simulink model "bit32mul"  (R2020a)
settings: Solver=VariableStepAuto  StartTime=0.0  StopTime=10.0  RelTol=1e-3
(part 37 of 50)

== system bit32mul/Subsystem1/Subsystem/Subsystem6/Subsystem/Subsystem5 ==
  In1 : Inport
  In2 : Inport  Port=2
  In3 : Inport  Port=3
  Logical Operator2 : Logic  Operator=XOR  AllPortsSameDT=off  OutDataTypeStr=boolean
  Logical Operator3 : Logic  Operator=XOR  AllPortsSameDT=off  OutDataTypeStr=boolean
  Out1 : Outport
  wires:
  In3/1 -> Logical Operator3/2
  In2/1 -> Logical Operator2/2
  In1/1 -> Logical Operator2/1
  Logical Operator2/1 -> Logical Operator3/1
  Logical Operator3/1 -> Out1/1

== system bit32mul/Subsystem1/Subsystem/Subsystem6/Subsystem/Subsystem6 ==
  In1 : Inport
  In2 : Inport  Port=2
  Logical Operator : Logic  Operator=XOR  AllPortsSameDT=off  OutDataTypeStr=boolean
  Logical Operator1 : Logic  AllPortsSameDT=off  OutDataTypeStr=boolean
  Out1 : Outport
  Out2 : Outport  Port=2
  wires:
  In1/1 -> Logical Operator1/1, Logical Operator/1
  Logical Operator1/1 -> Out2/1
  In2/1 -> Logical Operator1/2, Logical Operator/2
  Logical Operator/1 -> Out1/1

== system bit32mul/Subsystem1/Subsystem/Subsystem6/Subsystem/Subsystem7 ==
  In1 : Inport
  In2 : Inport  Port=2
  In3 : Inport  Port=3
  Logical Operator2 : Logic  Operator=XOR  AllPortsSameDT=off  OutDataTypeStr=boolean
  Logical Operator3 : Logic  Operator=XOR  AllPortsSameDT=off  OutDataTypeStr=boolean
  Out1 : Outport
  wires:
  In3/1 -> Logical Operator3/2
  In2/1 -> Logical Operator2/2
  In1/1 -> Logical Operator2/1
  Logical Operator2/1 -> Logical Operator3/1
  Logical Operator3/1 -> Out1/1

== system bit32mul/Subsystem1/Subsystem/Subsystem6/Subsystem/Subsystem8 ==
  In1 : Inport
  In2 : Inport  Port=2
  Logical Operator : Logic  Operator=XOR  AllPortsSameDT=off  OutDataTypeStr=boolean
  Logical Operator1 : Logic  AllPortsSameDT=off  OutDataTypeStr=boolean
  Out1 : Outport
  Out2 : Outport  Port=2
  wires:
  In1/1 -> Logical Operator1/1, Logical Operator/1
  Logical Operator1/1 -> Out2/1
  In2/1 -> Logical Operator1/2, Logical Operator/2
  Logical Operator/1 -> Out1/1

== system bit32mul/Subsystem1/Subsystem/Subsystem6/Subsystem4/Subsystem1 ==
  In1 : Inport
  In2 : Inport  Port=2
  Logical Operator : Logic  Operator=XOR  AllPortsSameDT=off  OutDataTypeStr=boolean
  Logical Operator1 : Logic  AllPortsSameDT=off  OutDataTypeStr=boolean
  Out1 : Outport
  Out2 : Outport  Port=2
  wires:
  In1/1 -> Logical Operator1/1, Logical Operator/1
  Logical Operator1/1 -> Out2/1
  In2/1 -> Logical Operator1/2, Logical Operator/2
  Logical Operator/1 -> Out1/1

== system bit32mul/Subsystem1/Subsystem/Subsystem6/Subsystem4/Subsystem2 ==
  In1 : Inport
  In2 : Inport  Port=2
  In3 : Inport  Port=3
  Logical Operator2 : Logic  Operator=XOR  AllPortsSameDT=off  OutDataTypeStr=boolean
  Logical Operator3 : Logic  Operator=XOR  AllPortsSameDT=off  OutDataTypeStr=boolean
  Out1 : Outport
  wires:
  In3/1 -> Logical Operator3/2
  In2/1 -> Logical Operator2/2
  In1/1 -> Logical Operator2/1
  Logical Operator2/1 -> Logical Operator3/1
  Logical Operator3/1 -> Out1/1

== system bit32mul/Subsystem1/Subsystem/Subsystem6/Subsystem4/Subsystem3 ==
  In1 : Inport
  In2 : Inport  Port=2
  In3 : Inport  Port=3
  Logical Operator2 : Logic  Operator=XOR  AllPortsSameDT=off  OutDataTypeStr=boolean
  Logical Operator3 : Logic  Operator=XOR  AllPortsSameDT=off  OutDataTypeStr=boolean
  Out1 : Outport
  wires:
  In3/1 -> Logical Operator3/2
  In2/1 -> Logical Operator2/2
  In1/1 -> Logical Operator2/1
  Logical Operator2/1 -> Logical Operator3/1
  Logical Operator3/1 -> Out1/1

== system bit32mul/Subsystem1/Subsystem/Subsystem6/Subsystem4/Subsystem4 ==
  In1 : Inport
  In2 : Inport  Port=2
  Logical Operator : Logic  Operator=XOR  AllPortsSameDT=off  OutDataTypeStr=boolean
  Logical Operator1 : Logic  AllPortsSameDT=off  OutDataTypeStr=boolean
  Out1 : Outport
  Out2 : Outport  Port=2
  wires:
  In1/1 -> Logical Operator1/1, Logical Operator/1
  Logical Operator1/1 -> Out2/1
  In2/1 -> Logical Operator1/2, Logical Operator/2
  Logical Operator/1 -> Out1/1

== system bit32mul/Subsystem1/Subsystem/Subsystem6/Subsystem4/Subsystem5 ==
  In1 : Inport
  In2 : Inport  Port=2
  In3 : Inport  Port=3
  Logical Operator2 : Logic  Operator=XOR  AllPortsSameDT=off  OutDataTypeStr=boolean
  Logical Operator3 : Logic  Operator=XOR  AllPortsSameDT=off  OutDataTypeStr=boolean
  Out1 : Outport
  wires:
  In3/1 -> Logical Operator3/2
  In2/1 -> Logical Operator2/2
  In1/1 -> Logical Operator2/1
  Logical Operator2/1 -> Logical Operator3/1
  Logical Operator3/1 -> Out1/1

== system bit32mul/Subsystem1/Subsystem/Subsystem6/Subsystem4/Subsystem6 ==
  In1 : Inport
  In2 : Inport  Port=2
  Logical Operator : Logic  Operator=XOR  AllPortsSameDT=off  OutDataTypeStr=boolean
  Logical Operator1 : Logic  AllPortsSameDT=off  OutDataTypeStr=boolean
  Out1 : Outport
  Out2 : Outport  Port=2
  wires:
  In1/1 -> Logical Operator1/1, Logical Operator/1
  Logical Operator1/1 -> Out2/1
  In2/1 -> Logical Operator1/2, Logical Operator/2
  Logical Operator/1 -> Out1/1

== system bit32mul/Subsystem1/Subsystem/Subsystem6/Subsystem4/Subsystem7 ==
  In1 : Inport
  In2 : Inport  Port=2
  In3 : Inport  Port=3
  Logical Operator2 : Logic  Operator=XOR  AllPortsSameDT=off  OutDataTypeStr=boolean
  Logical Operator3 : Logic  Operator=XOR  AllPortsSameDT=off  OutDataTypeStr=boolean
  Out1 : Outport
  wires:
  In3/1 -> Logical Operator3/2
  In2/1 -> Logical Operator2/2
  In1/1 -> Logical Operator2/1
  Logical Operator2/1 -> Logical Operator3/1
  Logical Operator3/1 -> Out1/1

== system bit32mul/Subsystem1/Subsystem/Subsystem6/Subsystem4/Subsystem8 ==
  In1 : Inport
  In2 : Inport  Port=2
  Logical Operator : Logic  Operator=XOR  AllPortsSameDT=off  OutDataTypeStr=boolean
  Logical Operator1 : Logic  AllPortsSameDT=off  OutDataTypeStr=boolean
  Out1 : Outport
  Out2 : Outport  Port=2
  wires:
  In1/1 -> Logical Operator1/1, Logical Operator/1
  Logical Operator1/1 -> Out2/1
  In2/1 -> Logical Operator1/2, Logical Operator/2
  Logical Operator/1 -> Out1/1

== system bit32mul/Subsystem1/Subsystem1/Subsystem4/Subsystem/Subsystem1 ==
  In1 : Inport
  In2 : Inport  Port=2
  Logical Operator : Logic  Operator=XOR  AllPortsSameDT=off  OutDataTypeStr=boolean
  Logical Operator1 : Logic  AllPortsSameDT=off  OutDataTypeStr=boolean
  Out1 : Outport
  Out2 : Outport  Port=2
  wires:
  In1/1 -> Logical Operator1/1, Logical Operator/1
  Logical Operator1/1 -> Out2/1
  In2/1 -> Logical Operator1/2, Logical Operator/2
  Logical Operator/1 -> Out1/1

== system bit32mul/Subsystem1/Subsystem1/Subsystem4/Subsystem/Subsystem2 ==
  In1 : Inport
  In2 : Inport  Port=2
  In3 : Inport  Port=3
  Logical Operator2 : Logic  Operator=XOR  AllPortsSameDT=off  OutDataTypeStr=boolean
  Logical Operator3 : Logic  Operator=XOR  AllPortsSameDT=off  OutDataTypeStr=boolean
  Out1 : Outport
  wires:
  In3/1 -> Logical Operator3/2
  In2/1 -> Logical Operator2/2
  In1/1 -> Logical Operator2/1
  Logical Operator2/1 -> Logical Operator3/1
  Logical Operator3/1 -> Out1/1

== system bit32mul/Subsystem1/Subsystem1/Subsystem4/Subsystem/Subsystem3 ==
  In1 : Inport
  In2 : Inport  Port=2
  In3 : Inport  Port=3
  Logical Operator2 : Logic  Operator=XOR  AllPortsSameDT=off  OutDataTypeStr=boolean
  Logical Operator3 : Logic  Operator=XOR  AllPortsSameDT=off  OutDataTypeStr=boolean
  Out1 : Outport
  wires:
  In3/1 -> Logical Operator3/2
  In2/1 -> Logical Operator2/2
  In1/1 -> Logical Operator2/1
  Logical Operator2/1 -> Logical Operator3/1
  Logical Operator3/1 -> Out1/1

== system bit32mul/Subsystem1/Subsystem1/Subsystem4/Subsystem/Subsystem4 ==
  In1 : Inport
  In2 : Inport  Port=2
  Logical Operator : Logic  Operator=XOR  AllPortsSameDT=off  OutDataTypeStr=boolean
  Logical Operator1 : Logic  AllPortsSameDT=off  OutDataTypeStr=boolean
  Out1 : Outport
  Out2 : Outport  Port=2
  wires:
  In1/1 -> Logical Operator1/1, Logical Operator/1
  Logical Operator1/1 -> Out2/1
  In2/1 -> Logical Operator1/2, Logical Operator/2
  Logical Operator/1 -> Out1/1

== system bit32mul/Subsystem1/Subsystem1/Subsystem4/Subsystem/Subsystem5 ==
  In1 : Inport
  In2 : Inport  Port=2
  In3 : Inport  Port=3
  Logical Operator2 : Logic  Operator=XOR  AllPortsSameDT=off  OutDataTypeStr=boolean
  Logical Operator3 : Logic  Operator=XOR  AllPortsSameDT=off  OutDataTypeStr=boolean
  Out1 : Outport
  wires:
  In3/1 -> Logical Operator3/2
  In2/1 -> Logical Operator2/2
  In1/1 -> Logical Operator2/1
  Logical Operator2/1 -> Logical Operator3/1
  Logical Operator3/1 -> Out1/1

== system bit32mul/Subsystem1/Subsystem1/Subsystem4/Subsystem/Subsystem6 ==
  In1 : Inport
  In2 : Inport  Port=2
  Logical Operator : Logic  Operator=XOR  AllPortsSameDT=off  OutDataTypeStr=boolean
  Logical Operator1 : Logic  AllPortsSameDT=off  OutDataTypeStr=boolean
  Out1 : Outport
  Out2 : Outport  Port=2
  wires:
  In1/1 -> Logical Operator1/1, Logical Operator/1
  Logical Operator1/1 -> Out2/1
  In2/1 -> Logical Operator1/2, Logical Operator/2
  Logical Operator/1 -> Out1/1

== system bit32mul/Subsystem1/Subsystem1/Subsystem4/Subsystem/Subsystem7 ==
  In1 : Inport
  In2 : Inport  Port=2
  In3 : Inport  Port=3
  Logical Operator2 : Logic  Operator=XOR  AllPortsSameDT=off  OutDataTypeStr=boolean
  Logical Operator3 : Logic  Operator=XOR  AllPortsSameDT=off  OutDataTypeStr=boolean
  Out1 : Outport
  wires:
  In3/1 -> Logical Operator3/2
  In2/1 -> Logical Operator2/2
  In1/1 -> Logical Operator2/1
  Logical Operator2/1 -> Logical Operator3/1
  Logical Operator3/1 -> Out1/1

== system bit32mul/Subsystem1/Subsystem1/Subsystem4/Subsystem/Subsystem8 ==
  In1 : Inport
  In2 : Inport  Port=2
  Logical Operator : Logic  Operator=XOR  AllPortsSameDT=off  OutDataTypeStr=boolean
  Logical Operator1 : Logic  AllPortsSameDT=off  OutDataTypeStr=boolean
  Out1 : Outport
  Out2 : Outport  Port=2
  wires:
  In1/1 -> Logical Operator1/1, Logical Operator/1
  Logical Operator1/1 -> Out2/1
  In2/1 -> Logical Operator1/2, Logical Operator/2
  Logical Operator/1 -> Out1/1

== system bit32mul/Subsystem1/Subsystem1/Subsystem4/Subsystem4/Subsystem1 ==
  In1 : Inport
  In2 : Inport  Port=2
  Logical Operator : Logic  Operator=XOR  AllPortsSameDT=off  OutDataTypeStr=boolean
  Logical Operator1 : Logic  AllPortsSameDT=off  OutDataTypeStr=boolean
  Out1 : Outport
  Out2 : Outport  Port=2
  wires:
  In1/1 -> Logical Operator1/1, Logical Operator/1
  Logical Operator1/1 -> Out2/1
  In2/1 -> Logical Operator1/2, Logical Operator/2
  Logical Operator/1 -> Out1/1

== system bit32mul/Subsystem1/Subsystem1/Subsystem4/Subsystem4/Subsystem2 ==
  In1 : Inport
  In2 : Inport  Port=2
  In3 : Inport  Port=3
  Logical Operator2 : Logic  Operator=XOR  AllPortsSameDT=off  OutDataTypeStr=boolean
  Logical Operator3 : Logic  Operator=XOR  AllPortsSameDT=off  OutDataTypeStr=boolean
  Out1 : Outport
  wires:
  In3/1 -> Logical Operator3/2
  In2/1 -> Logical Operator2/2
  In1/1 -> Logical Operator2/1
  Logical Operator2/1 -> Logical Operator3/1
  Logical Operator3/1 -> Out1/1

== system bit32mul/Subsystem1/Subsystem1/Subsystem4/Subsystem4/Subsystem3 ==
  In1 : Inport
  In2 : Inport  Port=2
  In3 : Inport  Port=3
  Logical Operator2 : Logic  Operator=XOR  AllPortsSameDT=off  OutDataTypeStr=boolean
  Logical Operator3 : Logic  Operator=XOR  AllPortsSameDT=off  OutDataTypeStr=boolean
  Out1 : Outport
  wires:
  In3/1 -> Logical Operator3/2
  In2/1 -> Logical Operator2/2
  In1/1 -> Logical Operator2/1
  Logical Operator2/1 -> Logical Operator3/1
  Logical Operator3/1 -> Out1/1

== system bit32mul/Subsystem1/Subsystem1/Subsystem4/Subsystem4/Subsystem4 ==
  In1 : Inport
  In2 : Inport  Port=2
  Logical Operator : Logic  Operator=XOR  AllPortsSameDT=off  OutDataTypeStr=boolean
  Logical Operator1 : Logic  AllPortsSameDT=off  OutDataTypeStr=boolean
  Out1 : Outport
  Out2 : Outport  Port=2
  wires:
  In1/1 -> Logical Operator1/1, Logical Operator/1
  Logical Operator1/1 -> Out2/1
  In2/1 -> Logical Operator1/2, Logical Operator/2
  Logical Operator/1 -> Out1/1

== system bit32mul/Subsystem1/Subsystem1/Subsystem4/Subsystem4/Subsystem5 ==
  In1 : Inport
  In2 : Inport  Port=2
  In3 : Inport  Port=3
  Logical Operator2 : Logic  Operator=XOR  AllPortsSameDT=off  OutDataTypeStr=boolean
  Logical Operator3 : Logic  Operator=XOR  AllPortsSameDT=off  OutDataTypeStr=boolean
  Out1 : Outport
  wires:
  In3/1 -> Logical Operator3/2
  In2/1 -> Logical Operator2/2
  In1/1 -> Logical Operator2/1
  Logical Operator2/1 -> Logical Operator3/1
  Logical Operator3/1 -> Out1/1

== system bit32mul/Subsystem1/Subsystem1/Subsystem4/Subsystem4/Subsystem6 ==
  In1 : Inport
  In2 : Inport  Port=2
  Logical Operator : Logic  Operator=XOR  AllPortsSameDT=off  OutDataTypeStr=boolean
  Logical Operator1 : Logic  AllPortsSameDT=off  OutDataTypeStr=boolean
  Out1 : Outport
  Out2 : Outport  Port=2
  wires:
  In1/1 -> Logical Operator1/1, Logical Operator/1
  Logical Operator1/1 -> Out2/1
  In2/1 -> Logical Operator1/2, Logical Operator/2
  Logical Operator/1 -> Out1/1

== system bit32mul/Subsystem1/Subsystem1/Subsystem4/Subsystem4/Subsystem7 ==
  In1 : Inport
  In2 : Inport  Port=2
  In3 : Inport  Port=3
  Logical Operator2 : Logic  Operator=XOR  AllPortsSameDT=off  OutDataTypeStr=boolean
  Logical Operator3 : Logic  Operator=XOR  AllPortsSameDT=off  OutDataTypeStr=boolean
  Out1 : Outport
  wires:
  In3/1 -> Logical Operator3/2
  In2/1 -> Logical Operator2/2
  In1/1 -> Logical Operator2/1
  Logical Operator2/1 -> Logical Operator3/1
  Logical Operator3/1 -> Out1/1

== system bit32mul/Subsystem1/Subsystem1/Subsystem4/Subsystem4/Subsystem8 ==
  In1 : Inport
  In2 : Inport  Port=2
  Logical Operator : Logic  Operator=XOR  AllPortsSameDT=off  OutDataTypeStr=boolean
  Logical Operator1 : Logic  AllPortsSameDT=off  OutDataTypeStr=boolean
  Out1 : Outport
  Out2 : Outport  Port=2
  wires:
  In1/1 -> Logical Operator1/1, Logical Operator/1
  Logical Operator1/1 -> Out2/1
  In2/1 -> Logical Operator1/2, Logical Operator/2
  Logical Operator/1 -> Out1/1

== system bit32mul/Subsystem1/Subsystem1/Subsystem5/Subsystem/Subsystem1 ==
  In1 : Inport
  In2 : Inport  Port=2
  Logical Operator : Logic  Operator=XOR  AllPortsSameDT=off  OutDataTypeStr=boolean
  Logical Operator1 : Logic  AllPortsSameDT=off  OutDataTypeStr=boolean
  Out1 : Outport
  Out2 : Outport  Port=2
  wires:
  In1/1 -> Logical Operator1/1, Logical Operator/1
  Logical Operator1/1 -> Out2/1
  In2/1 -> Logical Operator1/2, Logical Operator/2
  Logical Operator/1 -> Out1/1

== system bit32mul/Subsystem1/Subsystem1/Subsystem5/Subsystem/Subsystem2 ==
  In1 : Inport
  In2 : Inport  Port=2
  In3 : Inport  Port=3
  Logical Operator2 : Logic  Operator=XOR  AllPortsSameDT=off  OutDataTypeStr=boolean
  Logical Operator3 : Logic  Operator=XOR  AllPortsSameDT=off  OutDataTypeStr=boolean
  Out1 : Outport
  wires:
  In3/1 -> Logical Operator3/2
  In2/1 -> Logical Operator2/2
  In1/1 -> Logical Operator2/1
  Logical Operator2/1 -> Logical Operator3/1
  Logical Operator3/1 -> Out1/1

== system bit32mul/Subsystem1/Subsystem1/Subsystem5/Subsystem/Subsystem3 ==
  In1 : Inport
  In2 : Inport  Port=2
  In3 : Inport  Port=3
  Logical Operator2 : Logic  Operator=XOR  AllPortsSameDT=off  OutDataTypeStr=boolean
  Logical Operator3 : Logic  Operator=XOR  AllPortsSameDT=off  OutDataTypeStr=boolean
  Out1 : Outport
  wires:
  In3/1 -> Logical Operator3/2
  In2/1 -> Logical Operator2/2
  In1/1 -> Logical Operator2/1
  Logical Operator2/1 -> Logical Operator3/1
  Logical Operator3/1 -> Out1/1

== system bit32mul/Subsystem1/Subsystem1/Subsystem5/Subsystem/Subsystem4 ==
  In1 : Inport
  In2 : Inport  Port=2
  Logical Operator : Logic  Operator=XOR  AllPortsSameDT=off  OutDataTypeStr=boolean
  Logical Operator1 : Logic  AllPortsSameDT=off  OutDataTypeStr=boolean
  Out1 : Outport
  Out2 : Outport  Port=2
  wires:
  In1/1 -> Logical Operator1/1, Logical Operator/1
  Logical Operator1/1 -> Out2/1
  In2/1 -> Logical Operator1/2, Logical Operator/2
  Logical Operator/1 -> Out1/1

== system bit32mul/Subsystem1/Subsystem1/Subsystem5/Subsystem/Subsystem5 ==
  In1 : Inport
  In2 : Inport  Port=2
  In3 : Inport  Port=3
  Logical Operator2 : Logic  Operator=XOR  AllPortsSameDT=off  OutDataTypeStr=boolean
  Logical Operator3 : Logic  Operator=XOR  AllPortsSameDT=off  OutDataTypeStr=boolean
  Out1 : Outport
  wires:
  In3/1 -> Logical Operator3/2
  In2/1 -> Logical Operator2/2
  In1/1 -> Logical Operator2/1
  Logical Operator2/1 -> Logical Operator3/1
  Logical Operator3/1 -> Out1/1

== system bit32mul/Subsystem1/Subsystem1/Subsystem5/Subsystem/Subsystem6 ==
  In1 : Inport
  In2 : Inport  Port=2
  Logical Operator : Logic  Operator=XOR  AllPortsSameDT=off  OutDataTypeStr=boolean
  Logical Operator1 : Logic  AllPortsSameDT=off  OutDataTypeStr=boolean
  Out1 : Outport
  Out2 : Outport  Port=2
  wires:
  In1/1 -> Logical Operator1/1, Logical Operator/1
  Logical Operator1/1 -> Out2/1
  In2/1 -> Logical Operator1/2, Logical Operator/2
  Logical Operator/1 -> Out1/1

== system bit32mul/Subsystem1/Subsystem1/Subsystem5/Subsystem/Subsystem7 ==
  In1 : Inport
  In2 : Inport  Port=2
  In3 : Inport  Port=3
  Logical Operator2 : Logic  Operator=XOR  AllPortsSameDT=off  OutDataTypeStr=boolean
  Logical Operator3 : Logic  Operator=XOR  AllPortsSameDT=off  OutDataTypeStr=boolean
  Out1 : Outport
  wires:
  In3/1 -> Logical Operator3/2
  In2/1 -> Logical Operator2/2
  In1/1 -> Logical Operator2/1
  Logical Operator2/1 -> Logical Operator3/1
  Logical Operator3/1 -> Out1/1

== system bit32mul/Subsystem1/Subsystem1/Subsystem5/Subsystem/Subsystem8 ==
  In1 : Inport
  In2 : Inport  Port=2
  Logical Operator : Logic  Operator=XOR  AllPortsSameDT=off  OutDataTypeStr=boolean
  Logical Operator1 : Logic  AllPortsSameDT=off  OutDataTypeStr=boolean
  Out1 : Outport
  Out2 : Outport  Port=2
  wires:
  In1/1 -> Logical Operator1/1, Logical Operator/1
  Logical Operator1/1 -> Out2/1
  In2/1 -> Logical Operator1/2, Logical Operator/2
  Logical Operator/1 -> Out1/1

== system bit32mul/Subsystem1/Subsystem1/Subsystem5/Subsystem4/Subsystem1 ==
  In1 : Inport
  In2 : Inport  Port=2
  Logical Operator : Logic  Operator=XOR  AllPortsSameDT=off  OutDataTypeStr=boolean
  Logical Operator1 : Logic  AllPortsSameDT=off  OutDataTypeStr=boolean
  Out1 : Outport
  Out2 : Outport  Port=2
  wires:
  In1/1 -> Logical Operator1/1, Logical Operator/1
  Logical Operator1/1 -> Out2/1
  In2/1 -> Logical Operator1/2, Logical Operator/2
  Logical Operator/1 -> Out1/1

== system bit32mul/Subsystem1/Subsystem1/Subsystem5/Subsystem4/Subsystem2 ==
  In1 : Inport
  In2 : Inport  Port=2
  In3 : Inport  Port=3
  Logical Operator2 : Logic  Operator=XOR  AllPortsSameDT=off  OutDataTypeStr=boolean
  Logical Operator3 : Logic  Operator=XOR  AllPortsSameDT=off  OutDataTypeStr=boolean
  Out1 : Outport
  wires:
  In3/1 -> Logical Operator3/2
  In2/1 -> Logical Operator2/2
  In1/1 -> Logical Operator2/1
  Logical Operator2/1 -> Logical Operator3/1
  Logical Operator3/1 -> Out1/1

== system bit32mul/Subsystem1/Subsystem1/Subsystem5/Subsystem4/Subsystem3 ==
  In1 : Inport
  In2 : Inport  Port=2
  In3 : Inport  Port=3
  Logical Operator2 : Logic  Operator=XOR  AllPortsSameDT=off  OutDataTypeStr=boolean
  Logical Operator3 : Logic  Operator=XOR  AllPortsSameDT=off  OutDataTypeStr=boolean
  Out1 : Outport
  wires:
  In3/1 -> Logical Operator3/2
  In2/1 -> Logical Operator2/2
  In1/1 -> Logical Operator2/1
  Logical Operator2/1 -> Logical Operator3/1
  Logical Operator3/1 -> Out1/1

== system bit32mul/Subsystem1/Subsystem1/Subsystem5/Subsystem4/Subsystem4 ==
  In1 : Inport
  In2 : Inport  Port=2
  Logical Operator : Logic  Operator=XOR  AllPortsSameDT=off  OutDataTypeStr=boolean
  Logical Operator1 : Logic  AllPortsSameDT=off  OutDataTypeStr=boolean
  Out1 : Outport
  Out2 : Outport  Port=2
  wires:
  In1/1 -> Logical Operator1/1, Logical Operator/1
  Logical Operator1/1 -> Out2/1
  In2/1 -> Logical Operator1/2, Logical Operator/2
  Logical Operator/1 -> Out1/1

== system bit32mul/Subsystem1/Subsystem1/Subsystem5/Subsystem4/Subsystem5 ==
  In1 : Inport
  In2 : Inport  Port=2
  In3 : Inport  Port=3
  Logical Operator2 : Logic  Operator=XOR  AllPortsSameDT=off  OutDataTypeStr=boolean
  Logical Operator3 : Logic  Operator=XOR  AllPortsSameDT=off  OutDataTypeStr=boolean
  Out1 : Outport
  wires:
  In3/1 -> Logical Operator3/2
  In2/1 -> Logical Operator2/2
  In1/1 -> Logical Operator2/1
  Logical Operator2/1 -> Logical Operator3/1
  Logical Operator3/1 -> Out1/1

== system bit32mul/Subsystem1/Subsystem1/Subsystem5/Subsystem4/Subsystem6 ==
  In1 : Inport
  In2 : Inport  Port=2
  Logical Operator : Logic  Operator=XOR  AllPortsSameDT=off  OutDataTypeStr=boolean
  Logical Operator1 : Logic  AllPortsSameDT=off  OutDataTypeStr=boolean
  Out1 : Outport
  Out2 : Outport  Port=2
  wires:
  In1/1 -> Logical Operator1/1, Logical Operator/1
  Logical Operator1/1 -> Out2/1
  In2/1 -> Logical Operator1/2, Logical Operator/2
  Logical Operator/1 -> Out1/1

== system bit32mul/Subsystem1/Subsystem1/Subsystem5/Subsystem4/Subsystem7 ==
  In1 : Inport
  In2 : Inport  Port=2
  In3 : Inport  Port=3
  Logical Operator2 : Logic  Operator=XOR  AllPortsSameDT=off  OutDataTypeStr=boolean
  Logical Operator3 : Logic  Operator=XOR  AllPortsSameDT=off  OutDataTypeStr=boolean
  Out1 : Outport
  wires:
  In3/1 -> Logical Operator3/2
  In2/1 -> Logical Operator2/2
  In1/1 -> Logical Operator2/1
  Logical Operator2/1 -> Logical Operator3/1
  Logical Operator3/1 -> Out1/1

== system bit32mul/Subsystem1/Subsystem1/Subsystem5/Subsystem4/Subsystem8 ==
  In1 : Inport
  In2 : Inport  Port=2
  Logical Operator : Logic  Operator=XOR  AllPortsSameDT=off  OutDataTypeStr=boolean
  Logical Operator1 : Logic  AllPortsSameDT=off  OutDataTypeStr=boolean
  Out1 : Outport
  Out2 : Outport  Port=2
  wires:
  In1/1 -> Logical Operator1/1, Logical Operator/1
  Logical Operator1/1 -> Out2/1
  In2/1 -> Logical Operator1/2, Logical Operator/2
  Logical Operator/1 -> Out1/1

== system bit32mul/Subsystem1/Subsystem1/Subsystem6/Subsystem/Subsystem1 ==
  In1 : Inport
  In2 : Inport  Port=2
  Logical Operator : Logic  Operator=XOR  AllPortsSameDT=off  OutDataTypeStr=boolean
  Logical Operator1 : Logic  AllPortsSameDT=off  OutDataTypeStr=boolean
  Out1 : Outport
  Out2 : Outport  Port=2
  wires:
  In1/1 -> Logical Operator1/1, Logical Operator/1
  Logical Operator1/1 -> Out2/1
  In2/1 -> Logical Operator1/2, Logical Operator/2
  Logical Operator/1 -> Out1/1

== system bit32mul/Subsystem1/Subsystem1/Subsystem6/Subsystem/Subsystem2 ==
  In1 : Inport
  In2 : Inport  Port=2
  In3 : Inport  Port=3
  Logical Operator2 : Logic  Operator=XOR  AllPortsSameDT=off  OutDataTypeStr=boolean
  Logical Operator3 : Logic  Operator=XOR  AllPortsSameDT=off  OutDataTypeStr=boolean
  Out1 : Outport
  wires:
  In3/1 -> Logical Operator3/2
  In2/1 -> Logical Operator2/2
  In1/1 -> Logical Operator2/1
  Logical Operator2/1 -> Logical Operator3/1
  Logical Operator3/1 -> Out1/1

== system bit32mul/Subsystem1/Subsystem1/Subsystem6/Subsystem/Subsystem3 ==
  In1 : Inport
  In2 : Inport  Port=2
  In3 : Inport  Port=3
  Logical Operator2 : Logic  Operator=XOR  AllPortsSameDT=off  OutDataTypeStr=boolean
  Logical Operator3 : Logic  Operator=XOR  AllPortsSameDT=off  OutDataTypeStr=boolean
  Out1 : Outport
  wires:
  In3/1 -> Logical Operator3/2
  In2/1 -> Logical Operator2/2
  In1/1 -> Logical Operator2/1
  Logical Operator2/1 -> Logical Operator3/1
  Logical Operator3/1 -> Out1/1

== system bit32mul/Subsystem1/Subsystem1/Subsystem6/Subsystem/Subsystem4 ==
  In1 : Inport
  In2 : Inport  Port=2
  Logical Operator : Logic  Operator=XOR  AllPortsSameDT=off  OutDataTypeStr=boolean
  Logical Operator1 : Logic  AllPortsSameDT=off  OutDataTypeStr=boolean
  Out1 : Outport
  Out2 : Outport  Port=2
  wires:
  In1/1 -> Logical Operator1/1, Logical Operator/1
  Logical Operator1/1 -> Out2/1
  In2/1 -> Logical Operator1/2, Logical Operator/2
  Logical Operator/1 -> Out1/1

== system bit32mul/Subsystem1/Subsystem1/Subsystem6/Subsystem/Subsystem5 ==
  In1 : Inport
  In2 : Inport  Port=2
  In3 : Inport  Port=3
  Logical Operator2 : Logic  Operator=XOR  AllPortsSameDT=off  OutDataTypeStr=boolean
  Logical Operator3 : Logic  Operator=XOR  AllPortsSameDT=off  OutDataTypeStr=boolean
  Out1 : Outport
  wires:
  In3/1 -> Logical Operator3/2
  In2/1 -> Logical Operator2/2
  In1/1 -> Logical Operator2/1
  Logical Operator2/1 -> Logical Operator3/1
  Logical Operator3/1 -> Out1/1

== system bit32mul/Subsystem1/Subsystem1/Subsystem6/Subsystem/Subsystem6 ==
  In1 : Inport
  In2 : Inport  Port=2
  Logical Operator : Logic  Operator=XOR  AllPortsSameDT=off  OutDataTypeStr=boolean
  Logical Operator1 : Logic  AllPortsSameDT=off  OutDataTypeStr=boolean
  Out1 : Outport
  Out2 : Outport  Port=2
  wires:
  In1/1 -> Logical Operator1/1, Logical Operator/1
  Logical Operator1/1 -> Out2/1
  In2/1 -> Logical Operator1/2, Logical Operator/2
  Logical Operator/1 -> Out1/1

== system bit32mul/Subsystem1/Subsystem1/Subsystem6/Subsystem/Subsystem7 ==
  In1 : Inport
  In2 : Inport  Port=2
  In3 : Inport  Port=3
  Logical Operator2 : Logic  Operator=XOR  AllPortsSameDT=off  OutDataTypeStr=boolean
  Logical Operator3 : Logic  Operator=XOR  AllPortsSameDT=off  OutDataTypeStr=boolean
  Out1 : Outport
  wires:
  In3/1 -> Logical Operator3/2
  In2/1 -> Logical Operator2/2
  In1/1 -> Logical Operator2/1
  Logical Operator2/1 -> Logical Operator3/1
  Logical Operator3/1 -> Out1/1

== system bit32mul/Subsystem1/Subsystem1/Subsystem6/Subsystem/Subsystem8 ==
  In1 : Inport
  In2 : Inport  Port=2
  Logical Operator : Logic  Operator=XOR  AllPortsSameDT=off  OutDataTypeStr=boolean
  Logical Operator1 : Logic  AllPortsSameDT=off  OutDataTypeStr=boolean
  Out1 : Outport
  Out2 : Outport  Port=2
  wires:
  In1/1 -> Logical Operator1/1, Logical Operator/1
  Logical Operator1/1 -> Out2/1
  In2/1 -> Logical Operator1/2, Logical Operator/2
  Logical Operator/1 -> Out1/1

== system bit32mul/Subsystem1/Subsystem1/Subsystem6/Subsystem4/Subsystem1 ==
  In1 : Inport
  In2 : Inport  Port=2
  Logical Operator : Logic  Operator=XOR  AllPortsSameDT=off  OutDataTypeStr=boolean
  Logical Operator1 : Logic  AllPortsSameDT=off  OutDataTypeStr=boolean
  Out1 : Outport
  Out2 : Outport  Port=2
  wires:
  In1/1 -> Logical Operator1/1, Logical Operator/1
  Logical Operator1/1 -> Out2/1
  In2/1 -> Logical Operator1/2, Logical Operator/2
  Logical Operator/1 -> Out1/1

== system bit32mul/Subsystem1/Subsystem1/Subsystem6/Subsystem4/Subsystem2 ==
  In1 : Inport
  In2 : Inport  Port=2
  In3 : Inport  Port=3
  Logical Operator2 : Logic  Operator=XOR  AllPortsSameDT=off  OutDataTypeStr=boolean
  Logical Operator3 : Logic  Operator=XOR  AllPortsSameDT=off  OutDataTypeStr=boolean
  Out1 : Outport
  wires:
  In3/1 -> Logical Operator3/2
  In2/1 -> Logical Operator2/2
  In1/1 -> Logical Operator2/1
  Logical Operator2/1 -> Logical Operator3/1
  Logical Operator3/1 -> Out1/1

== system bit32mul/Subsystem1/Subsystem1/Subsystem6/Subsystem4/Subsystem3 ==
  In1 : Inport
  In2 : Inport  Port=2
  In3 : Inport  Port=3
  Logical Operator2 : Logic  Operator=XOR  AllPortsSameDT=off  OutDataTypeStr=boolean
  Logical Operator3 : Logic  Operator=XOR  AllPortsSameDT=off  OutDataTypeStr=boolean
  Out1 : Outport
  wires:
  In3/1 -> Logical Operator3/2
  In2/1 -> Logical Operator2/2
  In1/1 -> Logical Operator2/1
  Logical Operator2/1 -> Logical Operator3/1
  Logical Operator3/1 -> Out1/1

== system bit32mul/Subsystem1/Subsystem1/Subsystem6/Subsystem4/Subsystem4 ==
  In1 : Inport
  In2 : Inport  Port=2
  Logical Operator : Logic  Operator=XOR  AllPortsSameDT=off  OutDataTypeStr=boolean
  Logical Operator1 : Logic  AllPortsSameDT=off  OutDataTypeStr=boolean
  Out1 : Outport
  Out2 : Outport  Port=2
  wires:
  In1/1 -> Logical Operator1/1, Logical Operator/1
  Logical Operator1/1 -> Out2/1
  In2/1 -> Logical Operator1/2, Logical Operator/2
  Logical Operator/1 -> Out1/1

== system bit32mul/Subsystem1/Subsystem1/Subsystem6/Subsystem4/Subsystem5 ==
  In1 : Inport
  In2 : Inport  Port=2
  In3 : Inport  Port=3
  Logical Operator2 : Logic  Operator=XOR  AllPortsSameDT=off  OutDataTypeStr=boolean
  Logical Operator3 : Logic  Operator=XOR  AllPortsSameDT=off  OutDataTypeStr=boolean
  Out1 : Outport
  wires:
  In3/1 -> Logical Operator3/2
  In2/1 -> Logical Operator2/2
  In1/1 -> Logical Operator2/1
  Logical Operator2/1 -> Logical Operator3/1
  Logical Operator3/1 -> Out1/1

== system bit32mul/Subsystem1/Subsystem1/Subsystem6/Subsystem4/Subsystem6 ==
  In1 : Inport
  In2 : Inport  Port=2
  Logical Operator : Logic  Operator=XOR  AllPortsSameDT=off  OutDataTypeStr=boolean
  Logical Operator1 : Logic  AllPortsSameDT=off  OutDataTypeStr=boolean
  Out1 : Outport
  Out2 : Outport  Port=2
  wires:
  In1/1 -> Logical Operator1/1, Logical Operator/1
  Logical Operator1/1 -> Out2/1
  In2/1 -> Logical Operator1/2, Logical Operator/2
  Logical Operator/1 -> Out1/1

== system bit32mul/Subsystem1/Subsystem1/Subsystem6/Subsystem4/Subsystem7 ==
  In1 : Inport
  In2 : Inport  Port=2
  In3 : Inport  Port=3
  Logical Operator2 : Logic  Operator=XOR  AllPortsSameDT=off  OutDataTypeStr=boolean
  Logical Operator3 : Logic  Operator=XOR  AllPortsSameDT=off  OutDataTypeStr=boolean
  Out1 : Outport
  wires:
  In3/1 -> Logical Operator3/2
  In2/1 -> Logical Operator2/2
  In1/1 -> Logical Operator2/1
  Logical Operator2/1 -> Logical Operator3/1
  Logical Operator3/1 -> Out1/1

== system bit32mul/Subsystem1/Subsystem1/Subsystem6/Subsystem4/Subsystem8 ==
  In1 : Inport
  In2 : Inport  Port=2
  Logical Operator : Logic  Operator=XOR  AllPortsSameDT=off  OutDataTypeStr=boolean
  Logical Operator1 : Logic  AllPortsSameDT=off  OutDataTypeStr=boolean
  Out1 : Outport
  Out2 : Outport  Port=2
  wires:
  In1/1 -> Logical Operator1/1, Logical Operator/1
  Logical Operator1/1 -> Out2/1
  In2/1 -> Logical Operator1/2, Logical Operator/2
  Logical Operator/1 -> Out1/1

== system bit32mul/Subsystem1/Subsystem2/Subsystem4/Subsystem/Subsystem1 ==
  In1 : Inport
  In2 : Inport  Port=2
  Logical Operator : Logic  Operator=XOR  AllPortsSameDT=off  OutDataTypeStr=boolean
  Logical Operator1 : Logic  AllPortsSameDT=off  OutDataTypeStr=boolean
  Out1 : Outport
  Out2 : Outport  Port=2
  wires:
  In1/1 -> Logical Operator1/1, Logical Operator/1
  Logical Operator1/1 -> Out2/1
  In2/1 -> Logical Operator1/2, Logical Operator/2
  Logical Operator/1 -> Out1/1

== system bit32mul/Subsystem1/Subsystem2/Subsystem4/Subsystem/Subsystem2 ==
  In1 : Inport
  In2 : Inport  Port=2
  In3 : Inport  Port=3
  Logical Operator2 : Logic  Operator=XOR  AllPortsSameDT=off  OutDataTypeStr=boolean
  Logical Operator3 : Logic  Operator=XOR  AllPortsSameDT=off  OutDataTypeStr=boolean
  Out1 : Outport
  wires:
  In3/1 -> Logical Operator3/2
  In2/1 -> Logical Operator2/2
  In1/1 -> Logical Operator2/1
  Logical Operator2/1 -> Logical Operator3/1
  Logical Operator3/1 -> Out1/1

== system bit32mul/Subsystem1/Subsystem2/Subsystem4/Subsystem/Subsystem3 ==
  In1 : Inport
  In2 : Inport  Port=2
  In3 : Inport  Port=3
  Logical Operator2 : Logic  Operator=XOR  AllPortsSameDT=off  OutDataTypeStr=boolean
  Logical Operator3 : Logic  Operator=XOR  AllPortsSameDT=off  OutDataTypeStr=boolean
  Out1 : Outport
  wires:
  In3/1 -> Logical Operator3/2
  In2/1 -> Logical Operator2/2
  In1/1 -> Logical Operator2/1
  Logical Operator2/1 -> Logical Operator3/1
  Logical Operator3/1 -> Out1/1

== system bit32mul/Subsystem1/Subsystem2/Subsystem4/Subsystem/Subsystem4 ==
  In1 : Inport
  In2 : Inport  Port=2
  Logical Operator : Logic  Operator=XOR  AllPortsSameDT=off  OutDataTypeStr=boolean
  Logical Operator1 : Logic  AllPortsSameDT=off  OutDataTypeStr=boolean
  Out1 : Outport
  Out2 : Outport  Port=2
  wires:
  In1/1 -> Logical Operator1/1, Logical Operator/1
  Logical Operator1/1 -> Out2/1
  In2/1 -> Logical Operator1/2, Logical Operator/2
  Logical Operator/1 -> Out1/1

== system bit32mul/Subsystem1/Subsystem2/Subsystem4/Subsystem/Subsystem5 ==
  In1 : Inport
  In2 : Inport  Port=2
  In3 : Inport  Port=3
  Logical Operator2 : Logic  Operator=XOR  AllPortsSameDT=off  OutDataTypeStr=boolean
  Logical Operator3 : Logic  Operator=XOR  AllPortsSameDT=off  OutDataTypeStr=boolean
  Out1 : Outport
  wires:
  In3/1 -> Logical Operator3/2
  In2/1 -> Logical Operator2/2
  In1/1 -> Logical Operator2/1
  Logical Operator2/1 -> Logical Operator3/1
  Logical Operator3/1 -> Out1/1

== system bit32mul/Subsystem1/Subsystem2/Subsystem4/Subsystem/Subsystem6 ==
  In1 : Inport
  In2 : Inport  Port=2
  Logical Operator : Logic  Operator=XOR  AllPortsSameDT=off  OutDataTypeStr=boolean
  Logical Operator1 : Logic  AllPortsSameDT=off  OutDataTypeStr=boolean
  Out1 : Outport
  Out2 : Outport  Port=2
  wires:
  In1/1 -> Logical Operator1/1, Logical Operator/1
  Logical Operator1/1 -> Out2/1
  In2/1 -> Logical Operator1/2, Logical Operator/2
  Logical Operator/1 -> Out1/1

== system bit32mul/Subsystem1/Subsystem2/Subsystem4/Subsystem/Subsystem7 ==
  In1 : Inport
  In2 : Inport  Port=2
  In3 : Inport  Port=3
  Logical Operator2 : Logic  Operator=XOR  AllPortsSameDT=off  OutDataTypeStr=boolean
  Logical Operator3 : Logic  Operator=XOR  AllPortsSameDT=off  OutDataTypeStr=boolean
  Out1 : Outport
  wires:
  In3/1 -> Logical Operator3/2
  In2/1 -> Logical Operator2/2
  In1/1 -> Logical Operator2/1
  Logical Operator2/1 -> Logical Operator3/1
  Logical Operator3/1 -> Out1/1

== system bit32mul/Subsystem1/Subsystem2/Subsystem4/Subsystem/Subsystem8 ==
  In1 : Inport
  In2 : Inport  Port=2
  Logical Operator : Logic  Operator=XOR  AllPortsSameDT=off  OutDataTypeStr=boolean
  Logical Operator1 : Logic  AllPortsSameDT=off  OutDataTypeStr=boolean
  Out1 : Outport
  Out2 : Outport  Port=2
  wires:
  In1/1 -> Logical Operator1/1, Logical Operator/1
  Logical Operator1/1 -> Out2/1
  In2/1 -> Logical Operator1/2, Logical Operator/2
  Logical Operator/1 -> Out1/1

== system bit32mul/Subsystem1/Subsystem2/Subsystem4/Subsystem4/Subsystem1 ==
  In1 : Inport
  In2 : Inport  Port=2
  Logical Operator : Logic  Operator=XOR  AllPortsSameDT=off  OutDataTypeStr=boolean
  Logical Operator1 : Logic  AllPortsSameDT=off  OutDataTypeStr=boolean
  Out1 : Outport
  Out2 : Outport  Port=2
  wires:
  In1/1 -> Logical Operator1/1, Logical Operator/1
  Logical Operator1/1 -> Out2/1
  In2/1 -> Logical Operator1/2, Logical Operator/2
  Logical Operator/1 -> Out1/1

== system bit32mul/Subsystem1/Subsystem2/Subsystem4/Subsystem4/Subsystem2 ==
  In1 : Inport
  In2 : Inport  Port=2
  In3 : Inport  Port=3
  Logical Operator2 : Logic  Operator=XOR  AllPortsSameDT=off  OutDataTypeStr=boolean
  Logical Operator3 : Logic  Operator=XOR  AllPortsSameDT=off  OutDataTypeStr=boolean
  Out1 : Outport
  wires:
  In3/1 -> Logical Operator3/2
  In2/1 -> Logical Operator2/2
  In1/1 -> Logical Operator2/1
  Logical Operator2/1 -> Logical Operator3/1
  Logical Operator3/1 -> Out1/1

== system bit32mul/Subsystem1/Subsystem2/Subsystem4/Subsystem4/Subsystem3 ==
  In1 : Inport
  In2 : Inport  Port=2
  In3 : Inport  Port=3
  Logical Operator2 : Logic  Operator=XOR  AllPortsSameDT=off  OutDataTypeStr=boolean
  Logical Operator3 : Logic  Operator=XOR  AllPortsSameDT=off  OutDataTypeStr=boolean
  Out1 : Outport
  wires:
  In3/1 -> Logical Operator3/2
  In2/1 -> Logical Operator2/2
  In1/1 -> Logical Operator2/1
  Logical Operator2/1 -> Logical Operator3/1
  Logical Operator3/1 -> Out1/1

== system bit32mul/Subsystem1/Subsystem2/Subsystem4/Subsystem4/Subsystem4 ==
  In1 : Inport
  In2 : Inport  Port=2
  Logical Operator : Logic  Operator=XOR  AllPortsSameDT=off  OutDataTypeStr=boolean
  Logical Operator1 : Logic  AllPortsSameDT=off  OutDataTypeStr=boolean
  Out1 : Outport
  Out2 : Outport  Port=2
  wires:
  In1/1 -> Logical Operator1/1, Logical Operator/1
  Logical Operator1/1 -> Out2/1
  In2/1 -> Logical Operator1/2, Logical Operator/2
  Logical Operator/1 -> Out1/1

== system bit32mul/Subsystem1/Subsystem2/Subsystem4/Subsystem4/Subsystem5 ==
  In1 : Inport
  In2 : Inport  Port=2
  In3 : Inport  Port=3
  Logical Operator2 : Logic  Operator=XOR  AllPortsSameDT=off  OutDataTypeStr=boolean
  Logical Operator3 : Logic  Operator=XOR  AllPortsSameDT=off  OutDataTypeStr=boolean
  Out1 : Outport
  wires:
  In3/1 -> Logical Operator3/2
  In2/1 -> Logical Operator2/2
  In1/1 -> Logical Operator2/1
  Logical Operator2/1 -> Logical Operator3/1
  Logical Operator3/1 -> Out1/1

== system bit32mul/Subsystem1/Subsystem2/Subsystem4/Subsystem4/Subsystem6 ==
  In1 : Inport
  In2 : Inport  Port=2
  Logical Operator : Logic  Operator=XOR  AllPortsSameDT=off  OutDataTypeStr=boolean
  Logical Operator1 : Logic  AllPortsSameDT=off  OutDataTypeStr=boolean
  Out1 : Outport
  Out2 : Outport  Port=2
  wires:
  In1/1 -> Logical Operator1/1, Logical Operator/1
  Logical Operator1/1 -> Out2/1
  In2/1 -> Logical Operator1/2, Logical Operator/2
  Logical Operator/1 -> Out1/1

== system bit32mul/Subsystem1/Subsystem2/Subsystem4/Subsystem4/Subsystem7 ==
  In1 : Inport
  In2 : Inport  Port=2
  In3 : Inport  Port=3
  Logical Operator2 : Logic  Operator=XOR  AllPortsSameDT=off  OutDataTypeStr=boolean
  Logical Operator3 : Logic  Operator=XOR  AllPortsSameDT=off  OutDataTypeStr=boolean
  Out1 : Outport
  wires:
  In3/1 -> Logical Operator3/2
  In2/1 -> Logical Operator2/2
  In1/1 -> Logical Operator2/1
  Logical Operator2/1 -> Logical Operator3/1
  Logical Operator3/1 -> Out1/1

== system bit32mul/Subsystem1/Subsystem2/Subsystem4/Subsystem4/Subsystem8 ==
  In1 : Inport
  In2 : Inport  Port=2
  Logical Operator : Logic  Operator=XOR  AllPortsSameDT=off  OutDataTypeStr=boolean
  Logical Operator1 : Logic  AllPortsSameDT=off  OutDataTypeStr=boolean
  Out1 : Outport
  Out2 : Outport  Port=2
  wires:
  In1/1 -> Logical Operator1/1, Logical Operator/1
  Logical Operator1/1 -> Out2/1
  In2/1 -> Logical Operator1/2, Logical Operator/2
  Logical Operator/1 -> Out1/1

== system bit32mul/Subsystem1/Subsystem2/Subsystem5/Subsystem/Subsystem1 ==
  In1 : Inport
  In2 : Inport  Port=2
  Logical Operator : Logic  Operator=XOR  AllPortsSameDT=off  OutDataTypeStr=boolean
  Logical Operator1 : Logic  AllPortsSameDT=off  OutDataTypeStr=boolean
  Out1 : Outport
  Out2 : Outport  Port=2
  wires:
  In1/1 -> Logical Operator1/1, Logical Operator/1
  Logical Operator1/1 -> Out2/1
  In2/1 -> Logical Operator1/2, Logical Operator/2
  Logical Operator/1 -> Out1/1

== system bit32mul/Subsystem1/Subsystem2/Subsystem5/Subsystem/Subsystem2 ==
  In1 : Inport
  In2 : Inport  Port=2
  In3 : Inport  Port=3
  Logical Operator2 : Logic  Operator=XOR  AllPortsSameDT=off  OutDataTypeStr=boolean
  Logical Operator3 : Logic  Operator=XOR  AllPortsSameDT=off  OutDataTypeStr=boolean
  Out1 : Outport
  wires:
  In3/1 -> Logical Operator3/2
  In2/1 -> Logical Operator2/2
  In1/1 -> Logical Operator2/1
  Logical Operator2/1 -> Logical Operator3/1
  Logical Operator3/1 -> Out1/1

== system bit32mul/Subsystem1/Subsystem2/Subsystem5/Subsystem/Subsystem3 ==
  In1 : Inport
  In2 : Inport  Port=2
  In3 : Inport  Port=3
  Logical Operator2 : Logic  Operator=XOR  AllPortsSameDT=off  OutDataTypeStr=boolean
  Logical Operator3 : Logic  Operator=XOR  AllPortsSameDT=off  OutDataTypeStr=boolean
  Out1 : Outport
  wires:
  In3/1 -> Logical Operator3/2
  In2/1 -> Logical Operator2/2
  In1/1 -> Logical Operator2/1
  Logical Operator2/1 -> Logical Operator3/1
  Logical Operator3/1 -> Out1/1

== system bit32mul/Subsystem1/Subsystem2/Subsystem5/Subsystem/Subsystem4 ==
  In1 : Inport
  In2 : Inport  Port=2
  Logical Operator : Logic  Operator=XOR  AllPortsSameDT=off  OutDataTypeStr=boolean
  Logical Operator1 : Logic  AllPortsSameDT=off  OutDataTypeStr=boolean
  Out1 : Outport
  Out2 : Outport  Port=2
  wires:
  In1/1 -> Logical Operator1/1, Logical Operator/1
  Logical Operator1/1 -> Out2/1
  In2/1 -> Logical Operator1/2, Logical Operator/2
  Logical Operator/1 -> Out1/1

== system bit32mul/Subsystem1/Subsystem2/Subsystem5/Subsystem/Subsystem5 ==
  In1 : Inport
  In2 : Inport  Port=2
  In3 : Inport  Port=3
  Logical Operator2 : Logic  Operator=XOR  AllPortsSameDT=off  OutDataTypeStr=boolean
  Logical Operator3 : Logic  Operator=XOR  AllPortsSameDT=off  OutDataTypeStr=boolean
  Out1 : Outport
  wires:
  In3/1 -> Logical Operator3/2
  In2/1 -> Logical Operator2/2
  In1/1 -> Logical Operator2/1
  Logical Operator2/1 -> Logical Operator3/1
  Logical Operator3/1 -> Out1/1

== system bit32mul/Subsystem1/Subsystem2/Subsystem5/Subsystem/Subsystem6 ==
  In1 : Inport
  In2 : Inport  Port=2
  Logical Operator : Logic  Operator=XOR  AllPortsSameDT=off  OutDataTypeStr=boolean
  Logical Operator1 : Logic  AllPortsSameDT=off  OutDataTypeStr=boolean
  Out1 : Outport
  Out2 : Outport  Port=2
  wires:
  In1/1 -> Logical Operator1/1, Logical Operator/1
  Logical Operator1/1 -> Out2/1
  In2/1 -> Logical Operator1/2, Logical Operator/2
  Logical Operator/1 -> Out1/1

== system bit32mul/Subsystem1/Subsystem2/Subsystem5/Subsystem/Subsystem7 ==
  In1 : Inport
  In2 : Inport  Port=2
  In3 : Inport  Port=3
  Logical Operator2 : Logic  Operator=XOR  AllPortsSameDT=off  OutDataTypeStr=boolean
  Logical Operator3 : Logic  Operator=XOR  AllPortsSameDT=off  OutDataTypeStr=boolean
  Out1 : Outport
  wires:
  In3/1 -> Logical Operator3/2
  In2/1 -> Logical Operator2/2
  In1/1 -> Logical Operator2/1
  Logical Operator2/1 -> Logical Operator3/1
  Logical Operator3/1 -> Out1/1

== system bit32mul/Subsystem1/Subsystem2/Subsystem5/Subsystem/Subsystem8 ==
  In1 : Inport
  In2 : Inport  Port=2
  Logical Operator : Logic  Operator=XOR  AllPortsSameDT=off  OutDataTypeStr=boolean
  Logical Operator1 : Logic  AllPortsSameDT=off  OutDataTypeStr=boolean
  Out1 : Outport
  Out2 : Outport  Port=2
  wires:
  In1/1 -> Logical Operator1/1, Logical Operator/1
  Logical Operator1/1 -> Out2/1
  In2/1 -> Logical Operator1/2, Logical Operator/2
  Logical Operator/1 -> Out1/1

== system bit32mul/Subsystem1/Subsystem2/Subsystem5/Subsystem4/Subsystem1 ==
  In1 : Inport
  In2 : Inport  Port=2
  Logical Operator : Logic  Operator=XOR  AllPortsSameDT=off  OutDataTypeStr=boolean
  Logical Operator1 : Logic  AllPortsSameDT=off  OutDataTypeStr=boolean
  Out1 : Outport
  Out2 : Outport  Port=2
  wires:
  In1/1 -> Logical Operator1/1, Logical Operator/1
  Logical Operator1/1 -> Out2/1
  In2/1 -> Logical Operator1/2, Logical Operator/2
  Logical Operator/1 -> Out1/1

== system bit32mul/Subsystem1/Subsystem2/Subsystem5/Subsystem4/Subsystem2 ==
  In1 : Inport
  In2 : Inport  Port=2
  In3 : Inport  Port=3
  Logical Operator2 : Logic  Operator=XOR  AllPortsSameDT=off  OutDataTypeStr=boolean
  Logical Operator3 : Logic  Operator=XOR  AllPortsSameDT=off  OutDataTypeStr=boolean
  Out1 : Outport
  wires:
  In3/1 -> Logical Operator3/2
  In2/1 -> Logical Operator2/2
  In1/1 -> Logical Operator2/1
  Logical Operator2/1 -> Logical Operator3/1
  Logical Operator3/1 -> Out1/1

== system bit32mul/Subsystem1/Subsystem2/Subsystem5/Subsystem4/Subsystem3 ==
  In1 : Inport
  In2 : Inport  Port=2
  In3 : Inport  Port=3
  Logical Operator2 : Logic  Operator=XOR  AllPortsSameDT=off  OutDataTypeStr=boolean
  Logical Operator3 : Logic  Operator=XOR  AllPortsSameDT=off  OutDataTypeStr=boolean
  Out1 : Outport
  wires:
  In3/1 -> Logical Operator3/2
  In2/1 -> Logical Operator2/2
  In1/1 -> Logical Operator2/1
  Logical Operator2/1 -> Logical Operator3/1
  Logical Operator3/1 -> Out1/1

== system bit32mul/Subsystem1/Subsystem2/Subsystem5/Subsystem4/Subsystem4 ==
  In1 : Inport
  In2 : Inport  Port=2
  Logical Operator : Logic  Operator=XOR  AllPortsSameDT=off  OutDataTypeStr=boolean
  Logical Operator1 : Logic  AllPortsSameDT=off  OutDataTypeStr=boolean
  Out1 : Outport
  Out2 : Outport  Port=2
  wires:
  In1/1 -> Logical Operator1/1, Logical Operator/1
  Logical Operator1/1 -> Out2/1
  In2/1 -> Logical Operator1/2, Logical Operator/2
  Logical Operator/1 -> Out1/1

== system bit32mul/Subsystem1/Subsystem2/Subsystem5/Subsystem4/Subsystem5 ==
  In1 : Inport
  In2 : Inport  Port=2
  In3 : Inport  Port=3
  Logical Operator2 : Logic  Operator=XOR  AllPortsSameDT=off  OutDataTypeStr=boolean
  Logical Operator3 : Logic  Operator=XOR  AllPortsSameDT=off  OutDataTypeStr=boolean
  Out1 : Outport
  wires:
  In3/1 -> Logical Operator3/2
  In2/1 -> Logical Operator2/2
  In1/1 -> Logical Operator2/1
  Logical Operator2/1 -> Logical Operator3/1
  Logical Operator3/1 -> Out1/1

== system bit32mul/Subsystem1/Subsystem2/Subsystem5/Subsystem4/Subsystem6 ==
  In1 : Inport
  In2 : Inport  Port=2
  Logical Operator : Logic  Operator=XOR  AllPortsSameDT=off  OutDataTypeStr=boolean
  Logical Operator1 : Logic  AllPortsSameDT=off  OutDataTypeStr=boolean
  Out1 : Outport
  Out2 : Outport  Port=2
  wires:
  In1/1 -> Logical Operator1/1, Logical Operator/1
  Logical Operator1/1 -> Out2/1
  In2/1 -> Logical Operator1/2, Logical Operator/2
  Logical Operator/1 -> Out1/1

== system bit32mul/Subsystem1/Subsystem2/Subsystem5/Subsystem4/Subsystem7 ==
  In1 : Inport
  In2 : Inport  Port=2
  In3 : Inport  Port=3
  Logical Operator2 : Logic  Operator=XOR  AllPortsSameDT=off  OutDataTypeStr=boolean
  Logical Operator3 : Logic  Operator=XOR  AllPortsSameDT=off  OutDataTypeStr=boolean
  Out1 : Outport
  wires:
  In3/1 -> Logical Operator3/2
  In2/1 -> Logical Operator2/2
  In1/1 -> Logical Operator2/1
  Logical Operator2/1 -> Logical Operator3/1
  Logical Operator3/1 -> Out1/1

== system bit32mul/Subsystem1/Subsystem2/Subsystem5/Subsystem4/Subsystem8 ==
  In1 : Inport
  In2 : Inport  Port=2
  Logical Operator : Logic  Operator=XOR  AllPortsSameDT=off  OutDataTypeStr=boolean
  Logical Operator1 : Logic  AllPortsSameDT=off  OutDataTypeStr=boolean
  Out1 : Outport
  Out2 : Outport  Port=2
  wires:
  In1/1 -> Logical Operator1/1, Logical Operator/1
  Logical Operator1/1 -> Out2/1
  In2/1 -> Logical Operator1/2, Logical Operator/2
  Logical Operator/1 -> Out1/1

== system bit32mul/Subsystem1/Subsystem2/Subsystem6/Subsystem/Subsystem1 ==
  In1 : Inport
  In2 : Inport  Port=2
  Logical Operator : Logic  Operator=XOR  AllPortsSameDT=off  OutDataTypeStr=boolean
  Logical Operator1 : Logic  AllPortsSameDT=off  OutDataTypeStr=boolean
  Out1 : Outport
  Out2 : Outport  Port=2
  wires:
  In1/1 -> Logical Operator1/1, Logical Operator/1
  Logical Operator1/1 -> Out2/1
  In2/1 -> Logical Operator1/2, Logical Operator/2
  Logical Operator/1 -> Out1/1

== system bit32mul/Subsystem1/Subsystem2/Subsystem6/Subsystem/Subsystem2 ==
  In1 : Inport
  In2 : Inport  Port=2
  In3 : Inport  Port=3
  Logical Operator2 : Logic  Operator=XOR  AllPortsSameDT=off  OutDataTypeStr=boolean
  Logical Operator3 : Logic  Operator=XOR  AllPortsSameDT=off  OutDataTypeStr=boolean
  Out1 : Outport
  wires:
  In3/1 -> Logical Operator3/2
  In2/1 -> Logical Operator2/2
  In1/1 -> Logical Operator2/1
  Logical Operator2/1 -> Logical Operator3/1
  Logical Operator3/1 -> Out1/1

== system bit32mul/Subsystem1/Subsystem2/Subsystem6/Subsystem/Subsystem3 ==
  In1 : Inport
  In2 : Inport  Port=2
  In3 : Inport  Port=3
  Logical Operator2 : Logic  Operator=XOR  AllPortsSameDT=off  OutDataTypeStr=boolean
  Logical Operator3 : Logic  Operator=XOR  AllPortsSameDT=off  OutDataTypeStr=boolean
  Out1 : Outport
  wires:
  In3/1 -> Logical Operator3/2
  In2/1 -> Logical Operator2/2
  In1/1 -> Logical Operator2/1
  Logical Operator2/1 -> Logical Operator3/1
  Logical Operator3/1 -> Out1/1

== system bit32mul/Subsystem1/Subsystem2/Subsystem6/Subsystem/Subsystem4 ==
  In1 : Inport
  In2 : Inport  Port=2
  Logical Operator : Logic  Operator=XOR  AllPortsSameDT=off  OutDataTypeStr=boolean
  Logical Operator1 : Logic  AllPortsSameDT=off  OutDataTypeStr=boolean
  Out1 : Outport
  Out2 : Outport  Port=2
  wires:
  In1/1 -> Logical Operator1/1, Logical Operator/1
  Logical Operator1/1 -> Out2/1
  In2/1 -> Logical Operator1/2, Logical Operator/2
  Logical Operator/1 -> Out1/1

== system bit32mul/Subsystem1/Subsystem2/Subsystem6/Subsystem/Subsystem5 ==
  In1 : Inport
  In2 : Inport  Port=2
  In3 : Inport  Port=3
  Logical Operator2 : Logic  Operator=XOR  AllPortsSameDT=off  OutDataTypeStr=boolean
  Logical Operator3 : Logic  Operator=XOR  AllPortsSameDT=off  OutDataTypeStr=boolean
  Out1 : Outport
  wires:
  In3/1 -> Logical Operator3/2
  In2/1 -> Logical Operator2/2
  In1/1 -> Logical Operator2/1
  Logical Operator2/1 -> Logical Operator3/1
  Logical Operator3/1 -> Out1/1

== system bit32mul/Subsystem1/Subsystem2/Subsystem6/Subsystem/Subsystem6 ==
  In1 : Inport
  In2 : Inport  Port=2
  Logical Operator : Logic  Operator=XOR  AllPortsSameDT=off  OutDataTypeStr=boolean
  Logical Operator1 : Logic  AllPortsSameDT=off  OutDataTypeStr=boolean
  Out1 : Outport
  Out2 : Outport  Port=2
  wires:
  In1/1 -> Logical Operator1/1, Logical Operator/1
  Logical Operator1/1 -> Out2/1
  In2/1 -> Logical Operator1/2, Logical Operator/2
  Logical Operator/1 -> Out1/1

== system bit32mul/Subsystem1/Subsystem2/Subsystem6/Subsystem/Subsystem7 ==
  In1 : Inport
  In2 : Inport  Port=2
  In3 : Inport  Port=3
  Logical Operator2 : Logic  Operator=XOR  AllPortsSameDT=off  OutDataTypeStr=boolean
  Logical Operator3 : Logic  Operator=XOR  AllPortsSameDT=off  OutDataTypeStr=boolean
  Out1 : Outport
  wires:
  In3/1 -> Logical Operator3/2
  In2/1 -> Logical Operator2/2
  In1/1 -> Logical Operator2/1
  Logical Operator2/1 -> Logical Operator3/1
  Logical Operator3/1 -> Out1/1

== system bit32mul/Subsystem1/Subsystem2/Subsystem6/Subsystem/Subsystem8 ==
  In1 : Inport
  In2 : Inport  Port=2
  Logical Operator : Logic  Operator=XOR  AllPortsSameDT=off  OutDataTypeStr=boolean
  Logical Operator1 : Logic  AllPortsSameDT=off  OutDataTypeStr=boolean
  Out1 : Outport
  Out2 : Outport  Port=2
  wires:
  In1/1 -> Logical Operator1/1, Logical Operator/1
  Logical Operator1/1 -> Out2/1
  In2/1 -> Logical Operator1/2, Logical Operator/2
  Logical Operator/1 -> Out1/1
